simulink model "lab3_step_GM"  (R2020b)
settings: Solver=VariableStepAuto  StartTime=0.0  StopTime=10.0  RelTol=1e-3
values from neighbouring files (symbols this model uses):
  dc_gain = 3.26    [workspace.mat]
  k = 14.4844    [workspace.mat]
  p = 190    [workspace.mat]
  tau = 0.191    [workspace.mat]
  z = 48    [workspace.mat]
settings Model: Creator=MSI  LastModifiedBy=berksahin

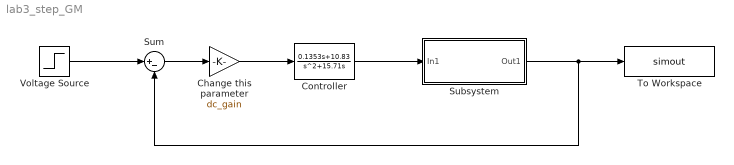
== system lab3_step_GM ==
  Change this parameter : Gain  Gain=dc_gain
  Controller : TransferFcn  Numerator=[0.1353 10.83]  Denominator=[1 15.71 0]
  Subsystem : Subsystem
  Sum : Sum  Inputs=|+-
  To Workspace : ToWorkspace  VariableName=simout  SaveFormat=Timeseries  SampleTime=-1
  Voltage Source : Step  Time=0  After=40  SampleTime=0
  wires:
  Voltage Source/1 -> Sum/1
  Sum/1 -> Change this parameter/1
  Change this parameter/1 -> Controller/1
  Controller/1 -> Subsystem/1(In1)
  Subsystem/1(Out1) -> Sum/2, To Workspace/1

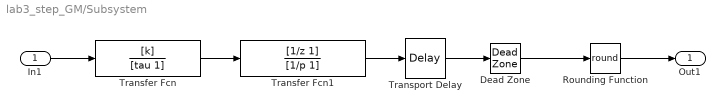
== system lab3_step_GM/Subsystem ==
  In1 : Inport
  Dead Zone : DeadZone  LowerValue=-5  UpperValue=5  SaturateOnIntegerOverflow=on
  Rounding Function : Rounding  Operator=round
  Transfer Fcn : TransferFcn  Numerator=[k]  Denominator=[tau 1]
  Transfer Fcn1 : TransferFcn  Numerator=[1/z 1]  Denominator=[1/p 1]
  Transport Delay : TransportDelay  DelayTime=0.01
  Out1 : Outport
  wires:
  Transfer Fcn/1 -> Transfer Fcn1/1
  In1/1 -> Transfer Fcn/1
  Rounding Function/1 -> Out1/1
  Transport Delay/1 -> Dead Zone/1
  Transfer Fcn1/1 -> Transport Delay/1
  Dead Zone/1 -> Rounding Function/1
